simulink model "tntc_closed_loop_sim"  (R2024a)
settings: Solver=VariableStepAuto  StartTime=0.0  StopTime=100  RelTol=1e-3
undefined symbols (not defined in the file): DiscIntNeverNeededParam
libraries: simulink x2
settings Model: Creator=ianmi  LastModifiedBy=ianmi

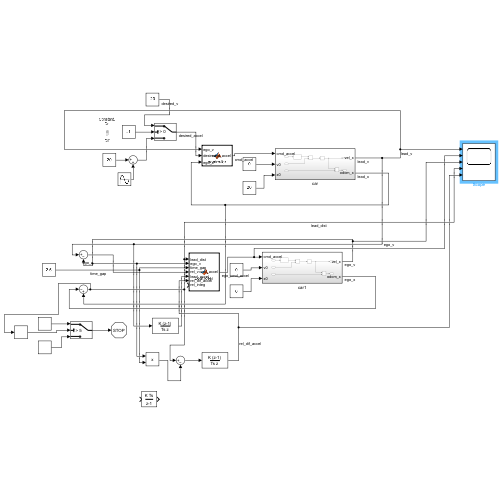
[thumbnail: Simulink's stored preview of the top-level diagram]
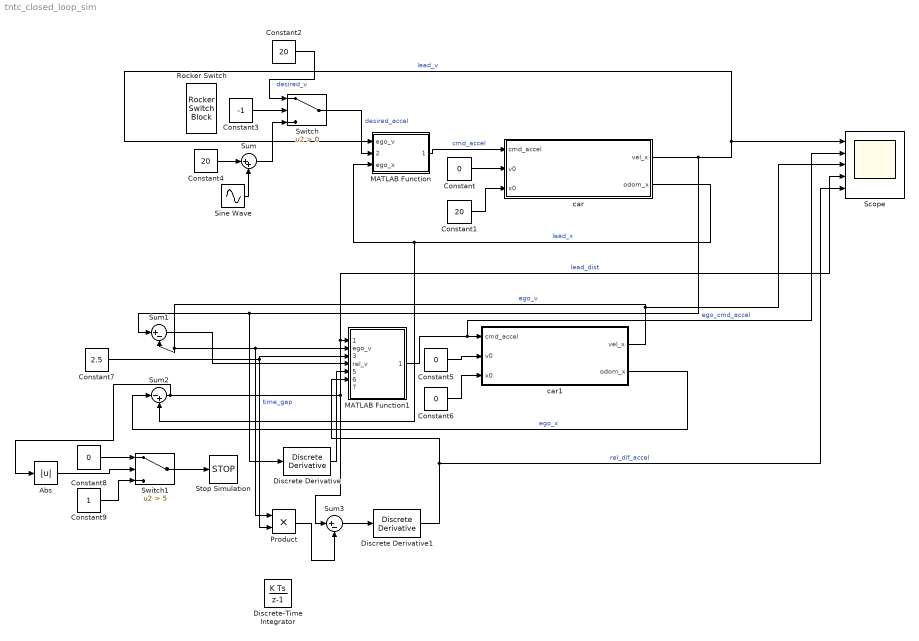
== system tntc_closed_loop_sim ==
  Abs : Abs  SaturateOnIntegerOverflow=off
  Constant{,5..6,8} (4 alike) : Constant  Value=0
  Constant1 : Constant  Value=20
  Constant2 : Constant  Value=20
  Constant3 : Constant  Value=-1
  Constant4 : Constant  Value=20
  Constant7 : Constant  Value=2.5
  Constant9 : Constant
  Discrete Derivative : simulink/Discrete/Discrete Derivative  gainval=1.0  ICPrevScaledInput=0.0  OutMin=[]  OutMax=[]  OutDataType=fixdt(1, 16)  OutScaling=2^-10  DoSatur=off
  Discrete Derivative1 : simulink/Discrete/Discrete Derivative  gainval=1.0  ICPrevScaledInput=0.0  OutMin=[]  OutMax=[]  OutDataType=fixdt(1, 16)  OutScaling=2^-10  DoSatur=off
  Discrete-Time Integrator : DiscreteIntegrator  SampleTime=-1  ICPrevOutput=DiscIntNeverNeededParam  ICPrevScaledInput=DiscIntNeverNeededParam
  MATLAB Function : MATLAB Function  TreatAsAtomicUnit=on
  MATLAB Function1 : MATLAB Function  TreatAsAtomicUnit=on
  Product : Product
  Rocker Switch : RockerSwitchBlock
      settings: Values={{'Off', 'On'}, [-1 1]}
  Scope : Scope  NumInputPorts=5
  Sine Wave : Sin  Amplitude=10  Frequency=0.5  SampleTime=0
  Stop Simulation : Stop
  Sum : Sum  Inputs=|++
  Sum1 : Sum  Inputs=|+-
  Sum2 : Sum  Inputs=|-+
  Sum3 : Sum  Inputs=|+-
  Switch : Switch  Criteria=u2 > Threshold  SaturateOnIntegerOverflow=off  InputSameDT=off
  Switch1 : Switch  Criteria=u2 > Threshold  Threshold=5  SaturateOnIntegerOverflow=off  InputSameDT=off
  car : Subsystem
  car1 : Subsystem
  wires:
  Constant3/1 -> Switch/2
  Constant4/1 -> Sum/1
  Switch/1 -> MATLAB Function/2(desired_v)  "desired_accel"
  Constant2/1 -> Switch/1  "desired_v"
  Sum/1 -> Switch/3
  car/1(vel_x) -> Discrete Derivative/1, Sum1/1, MATLAB Function/1(ego_v), Scope/1  "lead_v"
  car/2(odom_x) -> Sum2/2, MATLAB Function/3(ego_x)  "lead_x"
  MATLAB Function/1(cmd_accel) -> car/1(cmd_accel)  "cmd_accel"
  Constant/1 -> car/2(v0)
  Sine Wave/1 -> Sum/2
  Constant1/1 -> car/3(x0)
  Constant6/1 -> car1/3(x0)
  MATLAB Function1/1(cmd_accel) -> Scope/2, car1/1(cmd_accel)  "ego_cmd_accel"
  Constant5/1 -> car1/2(v0)
  car1/2(odom_x) -> Sum2/1  "ego_x"
  car1/1(vel_x) -> Scope/3, Sum1/2, MATLAB Function1/2(ego_v), Product/1  "ego_v"
  Sum1/1 -> MATLAB Function1/4(rel_v)
  Sum2/1 -> Scope/4, MATLAB Function1/1(lead_dist), Sum3/1, Abs/1  "lead_dist"
  Constant7/1 -> Product/2, MATLAB Function1/3(time_gap)  "time_gap"
  Constant8/1 -> Switch1/1
  Constant9/1 -> Switch1/3
  Abs/1 -> Switch1/2
  Switch1/1 -> Stop Simulation/1
  Discrete Derivative/1 -> MATLAB Function1/5(lead_accel)
  Product/1 -> Sum3/2
  Sum3/1 -> Discrete Derivative1/1
  Discrete Derivative1/1 -> Scope/5, MATLAB Function1/6(rel_dif_accel)  "rel_dif_accel"

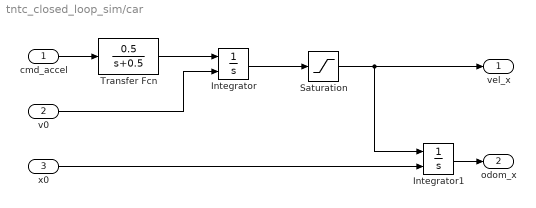
== system tntc_closed_loop_sim/car ==
  cmd_accel : Inport
  v0 : Inport  Port=2
  x0 : Inport  Port=3
  Integrator : Integrator  InitialConditionSource=external
  Integrator1 : Integrator  InitialConditionSource=external
  Saturation : Saturate  UpperLimit=80  LowerLimit=-80
  Transfer Fcn : TransferFcn  Numerator=[0.5]  Denominator=[1 0.5]
  vel_x : Outport
  odom_x : Outport  Port=2
  wires:
  v0/1 -> Integrator/2
  cmd_accel/1 -> Transfer Fcn/1
  Transfer Fcn/1 -> Integrator/1
  Integrator1/1 -> odom_x/1
  Integrator/1 -> Saturation/1
  x0/1 -> Integrator1/2
  Saturation/1 -> vel_x/1, Integrator1/1

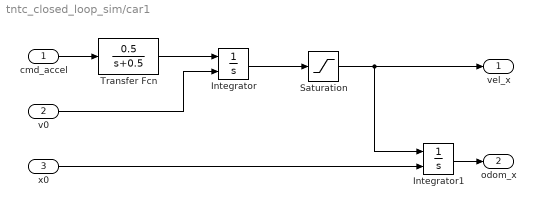
== system tntc_closed_loop_sim/car1 ==
  cmd_accel : Inport
  v0 : Inport  Port=2
  x0 : Inport  Port=3
  Integrator : Integrator  InitialConditionSource=external
  Integrator1 : Integrator  InitialConditionSource=external
  Saturation : Saturate  UpperLimit=80  LowerLimit=-80
  Transfer Fcn : TransferFcn  Numerator=[0.5]  Denominator=[1 0.5]
  vel_x : Outport
  odom_x : Outport  Port=2
  wires:
  v0/1 -> Integrator/2
  cmd_accel/1 -> Transfer Fcn/1
  Transfer Fcn/1 -> Integrator/1
  Integrator1/1 -> odom_x/1
  Integrator/1 -> Saturation/1
  x0/1 -> Integrator1/2
  Saturation/1 -> vel_x/1, Integrator1/1

== matlab function tntc_closed_loop_sim/MATLAB Function1 ==
  data: lead_dist input; ego_v input; time_gap input; rel_v input; cmd_accel output; lead_accel input; rel_dif_accel input; rel_integ input
function cmd_accel = controller(lead_dist, ego_v, time_gap, rel_v, lead_accel, rel_dif_accel, rel_integ)

force = 0.4

alpha = 0.4
beta = 1
gamma = 0.2
delta = 0.1

cmd_accel = alpha * (-ego_v * time_gap + lead_dist)
cmd_accel = cmd_accel + beta * lead_accel
cmd_accel = cmd_accel + gamma * rel_dif_accel
cmd_accel = cmd_accel + delta * rel_integ
cmd_accel = cmd_accel * force
if cmd_accel > 1.5
        cmd_accel = 1.5;
elseif cmd_accel < -3 
        cmd_accel = -3;
end

== matlab function tntc_closed_loop_sim/MATLAB Function ==
  data: ego_v input; desired_v input; cmd_accel output; ego_x input
function cmd_accel = controller(ego_v, desired_v, ego_x)

alpha = 0.3

cmd_accel = alpha * (desired_v - ego_v)
if cmd_accel > 1.5
        cmd_accel = 1.5;
elseif cmd_accel < -3 
        cmd_accel = -3;
end
